simulink model "CM620A_MotAg0Meas"  (R2013b)
settings: Solver=FixedStepDiscrete  SolverMode=SingleTasking  StartTime=0.0  StopTime=1  FixedStep=0.0000625  RelTol=1e-3
undefined symbols (not defined in the file): ARCHGLBPRM_2PI_ULS_F32, COEFFTBLELMSIZE_CNT_U08, COEFFTBLSIZE_CNT_U08, CORRNTBLAGSTEPSIZE_MATRAD_F32, CORRNTBLSIDXOFFS_CNT_U16, CORRNTBLSIZE_CNT_U16, CORRNTBLSIZEMASK_CNT_U08, FLTINJ_MOTAG0MEAS_MOTCTRLMOTAG0MECL, FLTINJ_MOTAG0MEAS_TESTOK, MotAg0PrtclFlt, MOTAG0PRTCLFLTFAILSTEP_CNT_U16, MOTAG0PRTCLFLTPASSSTEP_CNT_U16, MOTAGDELTAPERCORRNPT_CNT_U16, MOTAGIDXMASK_CNT_U16, MotCtrlMotAg0ErrReg, NtcSts1, sigbuilder_block, SNSRAGMASK_CNT_U32, SNSRERRMASK_CNT_U32, SNSRERRNTCMASK_CNT_U08, SNSRVLTGFLTMASK_CNT_U32, SPIPARMASK_CNT_U32
libraries: simulink x28, FloatToFixd x1, NxtrMax x1, NxtrLim x1
(part 2 of 4)

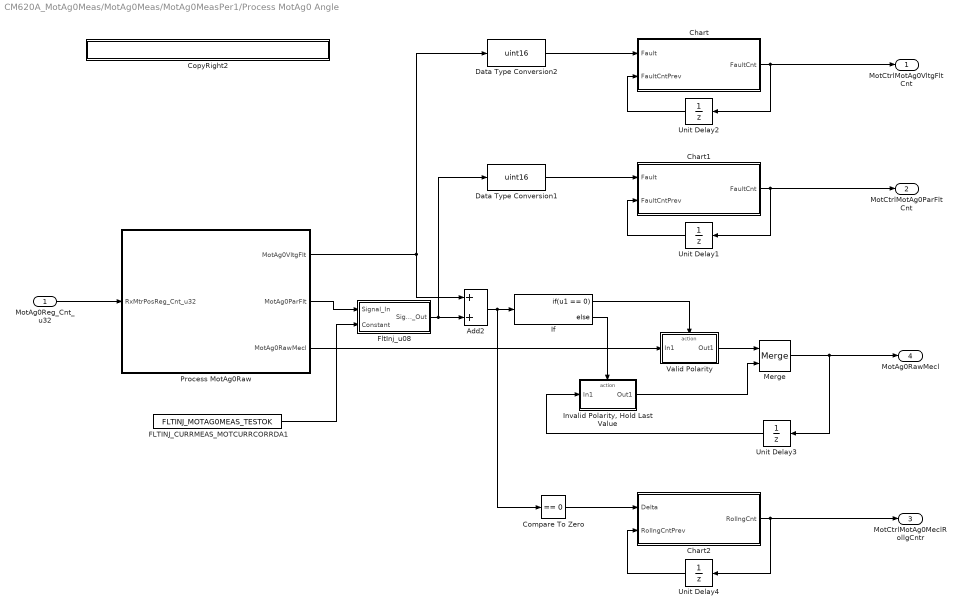
== system CM620A_MotAg0Meas/MotAg0Meas/MotAg0MeasPer1/Process MotAg0 Angle ==
  MotAg0Reg_Cnt_u32 : Inport
  Add2 : Sum  RequirementInfo={'linktype_rmi_doors' '0000c47b (/ESG Group/FDD Module Requirements/EA4 Specific/CM620A_MotAg0Meas)' '#CM620A_87' 'true' 'REQ: CM620A_87' '' } %GIDa_0b7de0f8_fdb6_403a_993a_161f92b64634
  Chart : Stateflow chart  TreatAsAtomicUnit=on
  Chart1 : Stateflow chart  TreatAsAtomicUnit=on
  Chart2 : Stateflow chart  RequirementInfo={'linktype_rmi_doors' '0000c47b (/ESG Group/FDD Module Requirements/EA4 Specific/CM620A_MotAg0Meas)' '#CM620A_107' 'true' 'REQ: CM620A_107' '' } %GIDa_4e204d7d_fe00_4721_af4a_71a94d72e207  TreatAsAtomicUnit=on
  Compare To Zero : simulink/Logic and Bit Operations/Compare To Zero  relop===  OutDataTypeStr=uint8
  CopyRight2 : Subsystem  Description=|  mask(Copyright Information){none=on}
      | Copyright info block.                                               
      |                                                                     
      | Place copyright information at the top of every subsystem in design.
      mask prompts: none "No parameters"
      mask help: Place copyright information at the top of every subsystem in design.
      mask Display:
      | NxtrConf = 'Nexteer Confidential';
      | 
      | sys = bdroot; %handle for the current model ("system")
      | first = get_param(sys,'Created');
      | first = first(end-3:end);  %year is last four digits
      | 
      | last = get_param(sys,'LastModifiedDate');
      | if isempty(last)
      |     last = datestr(now,'yyyy');
      | else
      |     last = last(end-3:end);
      | end
      | 
      | if strcmp(first,last)
      |     fprintf('%s -- Copyright %s Nexteer',NxtrConf,first)
      | else
      |     fprintf('%s -- %s%s- %s Nexteer',NxtrConf,char(169),first,last)
      | end
  Data Type Conversion1 : DataTypeConversion  OutDataTypeStr=uint16
  Data Type Conversion2 : DataTypeConversion  OutDataTypeStr=uint16
  FLTINJ_CURRMEAS_MOTCURRCORRDA1 : Constant  Value=FLTINJ_MOTAG0MEAS_TESTOK
  FltInj_u08 : Subsystem  RequirementInfo={'linktype_rmi_doors' '0000c47b (/ESG Group/FDD Module Requirements/EA4 Specific/CM620A_MotAg0Meas)' '#CM620A_111' 'true' 'REQ: CM620A_111' '' } %GIDa_ea97dbee_e66e_4906_919b_b7ed9fef212d  TreatAsAtomicUnit=on  VariantControl=FltInj_sim  mask(Fault_Injection){}
      mask help: Fault Injection is a simulation only block for EA3 programs.
  If : If  IfExpression=u1 == 0
  "Invalid Polarity, Hold Last Value" : Subsystem  TreatAsAtomicUnit=on
  Merge : Merge  RequirementInfo={'linktype_rmi_doors' '0000c47b (/ESG Group/FDD Module Requirements/EA4 Specific/CM620A_MotAg0Meas)' '#CM620A_88' 'true' 'REQ: CM620A_88' '' } %GIDa_2a6c3b81_7733_45e8_b94f_934422d25578
  Process MotAg0Raw : Subsystem  RequirementInfo={'linktype_rmi_doors' '0000c47b (/ESG Group/FDD Module Requirements/EA4 Specific/CM620A_MotAg0Meas)' '#CM620A_95' 'true' 'REQ: CM620A_95' '' ; 'linktype_rmi_doors' '0000c47b (/ESG Group/FDD Module Requirements/EA4 Specific/CM620A_MotAg0Meas)' '#CM620A_93' 'true' 'REQ: CM620A_93' '' ; 'linktype_rmi_doors' '0000c47b (/ESG Group/FDD Module Requirements/EA4 Specific/CM620A_MotAg0Meas)' '#CM620A_84' 'true' 'REQ: CM620A_84' '' ; 'linktype_rmi_doors' '0000c47b (/ESG Group/FDD Module Requirements/EA4 Specific/CM620A_MotAg0Meas)' '#CM620A_86' 'true' 'REQ: CM620A_86' '' } %GIDa_f2e2859c_06d0_4da9_b7a1_6837a8f50074
  Unit Delay1 : UnitDelay  SampleTime=-1  StateName=MotAg0ParFltCntPrev  StateMustResolveToSignalObject=on
      settings: AttributesFormatString=|
      | State Variable:
      | %<StateName>
  Unit Delay2 : UnitDelay  SampleTime=-1  StateName=MotAg0VltgFltCntPrev  StateMustResolveToSignalObject=on
      settings: AttributesFormatString=|
      | State Variable:
      | %<StateName>
  Unit Delay3 : UnitDelay  SampleTime=-1  StateName=MotAg0RawMeclPrev  StateMustResolveToSignalObject=on
      settings: AttributesFormatString=|
      | State Variable:
      | %<StateName>
  Unit Delay4 : UnitDelay  SampleTime=-1  StateName=MotAg0MeclRollgCntrPrev  StateMustResolveToSignalObject=on
      settings: AttributesFormatString=|
      | State Variable:
      | %<StateName>
  Valid Polarity : Subsystem  TreatAsAtomicUnit=on
  MotCtrlMotAg0VltgFltCnt : Outport
  MotCtrlMotAg0ParFltCnt : Outport  Port=2
  MotCtrlMotAg0MeclRollgCntr : Outport  Port=3
  MotAg0RawMecl : Outport  Port=4
  wires:
  Add2/1 -> If/1, Compare To Zero/1
  Process MotAg0Raw/1(MotAg0VltgFlt) -> Data Type Conversion2/1, Add2/1
  Unit Delay3/1 -> "Invalid Polarity, Hold Last Value"/1(In1)
  Merge/1 -> Unit Delay3/1, MotAg0RawMecl/1
  MotAg0Reg_Cnt_u32/1 -> Process MotAg0Raw/1(RxMtrPosReg_Cnt_u32)
  "Invalid Polarity, Hold Last Value"/1(Out1) -> Merge/2
  Valid Polarity/1(Out1) -> Merge/1
  If/2 -> "Invalid Polarity, Hold Last Value"/Action
  If/1 -> Valid Polarity/Action
  Process MotAg0Raw/3(MotAg0RawMecl) -> Valid Polarity/1(In1)
  Data Type Conversion2/1 -> Chart/1(Fault)
  Chart/1(FaultCnt) -> MotCtrlMotAg0VltgFltCnt/1, Unit Delay2/1
  Unit Delay2/1 -> Chart/2(FaultCntPrev)
  Data Type Conversion1/1 -> Chart1/1(Fault)
  Chart1/1(FaultCnt) -> MotCtrlMotAg0ParFltCnt/1, Unit Delay1/1
  Unit Delay1/1 -> Chart1/2(FaultCntPrev)
  Compare To Zero/1 -> Chart2/1(Delta)
  Chart2/1(RollngCnt) -> MotCtrlMotAg0MeclRollgCntr/1, Unit Delay4/1
  Unit Delay4/1 -> Chart2/2(RollngCntPrev)
  FLTINJ_CURRMEAS_MOTCURRCORRDA1/1 -> FltInj_u08/2(Constant)
  Process MotAg0Raw/2(MotAg0ParFlt) -> FltInj_u08/1(Signal_In)
  FltInj_u08/1(Signal_Out) -> Add2/2, Data Type Conversion1/1

== system CM620A_MotAg0Meas/MotAg0Meas/MotAg0MeasPer2/CopyRight2 ==

== system CM620A_MotAg0Meas/MotAg0Meas/MotAg0MeasPer2/MotAg0 Protocol Fault Operation ==
  note: Function Call Sequence Requirements
      |
      | - GetNtcQlfr shall execute after SetNtcSts
  MotAg0Err : Inport
  MotAg0ErrParFltCnt : Inport  Port=2
  MotAg0ParFltCnt : Inport  Port=3
  MotAg0VltgFltCnt : Inport  Port=4
  Atomic Subsystem : Subsystem  TreatAsAtomicUnit=on
  Constant3 : Constant  Value=MotAg0PrtclFlt
  CopyRight2 : Subsystem  Description=|  mask(Copyright Information){none=on}
      | Copyright info block.                                               
      |                                                                     
      | Place copyright information at the top of every subsystem in design.
      mask prompts: none "No parameters"
      mask help: Place copyright information at the top of every subsystem in design.
      mask Display:
      | NxtrConf = 'Nexteer Confidential';
      | 
      | sys = bdroot; %handle for the current model ("system")
      | first = get_param(sys,'Created');
      | first = first(end-3:end);  %year is last four digits
      | 
      | last = get_param(sys,'LastModifiedDate');
      | if isempty(last)
      |     last = datestr(now,'yyyy');
      | else
      |     last = last(end-3:end);
      | end
      | 
      | if strcmp(first,last)
      |     fprintf('%s -- Copyright %s Nexteer',NxtrConf,first)
      | else
      |     fprintf('%s -- %s%s- %s Nexteer',NxtrConf,char(169),first,last)
      | end
  Data store for model purposes only - don't code : DataStoreMemory  DataStoreName=NtcQlfr  ReadBeforeWriteMsg=warning  WriteAfterWriteMsg=warning  WriteAfterReadMsg=warning
  GetNtcQlfr : Subsystem  RequirementInfo={'linktype_rmi_doors' '0000c47b (/ESG Group/FDD Module Requirements/EA4 Specific/CM620A_MotAg0Meas)' '#CM620A_106' 'true' 'REQ: CM620A_106' '' } %GIDa_2788174b_a957_4dc9_a642_eff6dc86ed2e
  SetNtcSts : Subsystem
  Subsystem : Subsystem
  MotAg0Qlfr : Outport  RequirementInfo={} %GIDa_cf1cbe4f_1681_476d_80fb_f928627be900
  wires:
  MotAg0Err/1 -> Subsystem/1(MotAg0Err)
  MotAg0ErrParFltCnt/1 -> Subsystem/2(MotAg0ErrParFltCnt)
  MotAg0ParFltCnt/1 -> Subsystem/3(MotAg0ParFltCnt)
  MotAg0VltgFltCnt/1 -> Subsystem/4(MotAg0VltgFltCnt)
  Constant3/1 -> SetNtcSts/1(NtcNr), GetNtcQlfr/1(NtcNr)  "NtcNr"
  GetNtcQlfr/1(NtcQlfr) -> MotAg0Qlfr/1
  Atomic Subsystem/1(NtcSts) -> SetNtcSts/3(NtcSts)
  Atomic Subsystem/2(DebStep) -> SetNtcSts/4(DebStep)
  Subsystem/1(NtcStInfo) -> Atomic Subsystem/1(NtcStInfo), SetNtcSts/2(NtcStInfo)  "ParamByte"

== system CM620A_MotAg0Meas/MotAg0Meas/MotAg0MeasPer2/Process ErrorReg and DieRevCtr ==
  MotAg0ErrReg : Inport  OutDataTypeStr=uint32
  CopyRight2 : Subsystem  Description=|  mask(Copyright Information){none=on}
      | Copyright info block.                                               
      |                                                                     
      | Place copyright information at the top of every subsystem in design.
      mask prompts: none "No parameters"
      mask help: Place copyright information at the top of every subsystem in design.
      mask Display:
      | NxtrConf = 'Nexteer Confidential';
      | 
      | sys = bdroot; %handle for the current model ("system")
      | first = get_param(sys,'Created');
      | first = first(end-3:end);  %year is last four digits
      | 
      | last = get_param(sys,'LastModifiedDate');
      | if isempty(last)
      |     last = datestr(now,'yyyy');
      | else
      |     last = last(end-3:end);
      | end
      | 
      | if strcmp(first,last)
      |     fprintf('%s -- Copyright %s Nexteer',NxtrConf,first)
      | else
      |     fprintf('%s -- %s%s- %s Nexteer',NxtrConf,char(169),first,last)
      | end
  Process MotAg0RawErr : Subsystem  RequirementInfo={'linktype_rmi_doors' '0000c47b (/ESG Group/FDD Module Requirements/EA4 Specific/CM620A_MotAg0Meas)' '#CM620A_93' 'true' 'REQ: CM620A_93' '' } %GIDa_05fef35d_e67f_443b_a4d0_6048385f8050
  MotAg0Err : Outport  OutDataTypeStr=uint8
  MotAg0ErrParFltCnt : Outport  Port=2
  wires:
  MotAg0ErrReg/1 -> Process MotAg0RawErr/1(MotAg0ErrReg)
  Process MotAg0RawErr/1(MotAg0ErrParFltCnt) -> MotAg0ErrParFltCnt/1
  Process MotAg0RawErr/2(MotAg0Err) -> MotAg0Err/1

== system CM620A_MotAg0Meas/MotAg0Meas/MotAg0MeasInit1/Compute Correction Table/CopyRight2 ==

== system CM620A_MotAg0Meas/MotAg0Meas/MotAg0MeasInit1/Compute Correction Table/MotAg0CoeffTbl_GetErrorStatus ==
  note: 0 simulated for modeling purposes,
      | actual value returned by NVM.  Non-zero return indicates
      | failure in storage/retrievial of NVM.
  Constant : Constant  Value=0
  CopyRight2 : Subsystem  Description=|  mask(Copyright Information){none=on}
      | Copyright info block.                                               
      |                                                                     
      | Place copyright information at the top of every subsystem in design.
      mask prompts: none "No parameters"
      mask help: Place copyright information at the top of every subsystem in design.
      mask Display:
      | NxtrConf = 'Nexteer Confidential';
      | 
      | sys = bdroot; %handle for the current model ("system")
      | first = get_param(sys,'Created');
      | first = first(end-3:end);  %year is last four digits
      | 
      | last = get_param(sys,'LastModifiedDate');
      | if isempty(last)
      |     last = datestr(now,'yyyy');
      | else
      |     last = last(end-3:end);
      | end
      | 
      | if strcmp(first,last)
      |     fprintf('%s -- Copyright %s Nexteer',NxtrConf,first)
      | else
      |     fprintf('%s -- %s%s- %s Nexteer',NxtrConf,char(169),first,last)
      | end
  RequestResultPtr : Outport
  wires:
  Constant/1 -> RequestResultPtr/1

== system CM620A_MotAg0Meas/MotAg0Meas/MotAg0MeasInit1/Compute Correction Table/NVM NOK ==
  note: In the event of a NVM failure
      | set the correction table to 0
  Action Port : ActionPort  ActionType=else
  Constant1 : Constant  Value=CORRNTBLSIZE_CNT_U16
  CopyRight2 : Subsystem  Description=|  mask(Copyright Information){none=on}
      | Copyright info block.                                               
      |                                                                     
      | Place copyright information at the top of every subsystem in design.
      mask prompts: none "No parameters"
      mask help: Place copyright information at the top of every subsystem in design.
      mask Display:
      | NxtrConf = 'Nexteer Confidential';
      | 
      | sys = bdroot; %handle for the current model ("system")
      | first = get_param(sys,'Created');
      | first = first(end-3:end);  %year is last four digits
      | 
      | last = get_param(sys,'LastModifiedDate');
      | if isempty(last)
      |     last = datestr(now,'yyyy');
      | else
      |     last = last(end-3:end);
      | end
      | 
      | if strcmp(first,last)
      |     fprintf('%s -- Copyright %s Nexteer',NxtrConf,first)
      | else
      |     fprintf('%s -- %s%s- %s Nexteer',NxtrConf,char(169),first,last)
      | end
  Zero out correction table : Subsystem  TreatAsAtomicUnit=on
  wires:
  Constant1/1 -> Zero out correction table/1(N)

== system CM620A_MotAg0Meas/MotAg0Meas/MotAg0MeasInit1/Compute Correction Table/NVM Ok ==
  Action Port : ActionPort  ActionType=then
  Calculate Correction Table : Subsystem  Priority=100  TreatAsAtomicUnit=on
      settings: AttributesFormatString=|
      | Priority:
      | %<Priority>
  Configure Coefficients : Subsystem  Priority=10  TreatAsAtomicUnit=on
      settings: AttributesFormatString=|
      | Priority:
      | %<Priority>
  CopyRight2 : Subsystem  Description=|  mask(Copyright Information){none=on}
      | Copyright info block.                                               
      |                                                                     
      | Place copyright information at the top of every subsystem in design.
      mask prompts: none "No parameters"
      mask help: Place copyright information at the top of every subsystem in design.
      mask Display:
      | NxtrConf = 'Nexteer Confidential';
      | 
      | sys = bdroot; %handle for the current model ("system")
      | first = get_param(sys,'Created');
      | first = first(end-3:end);  %year is last four digits
      | 
      | last = get_param(sys,'LastModifiedDate');
      | if isempty(last)
      |     last = datestr(now,'yyyy');
      | else
      |     last = last(end-3:end);
      | end
      | 
      | if strcmp(first,last)
      |     fprintf('%s -- Copyright %s Nexteer',NxtrConf,first)
      | else
      |     fprintf('%s -- %s%s- %s Nexteer',NxtrConf,char(169),first,last)
      | end

== system CM620A_MotAg0Meas/MotAg0Meas/MotAg0MeasInit1/Initialize CSIH Registers/CopyRight2 ==

== system CM620A_MotAg0Meas/MotAg0Meas/MotAg0MeasPer1/Compensate MechMtrPos1/CopyRight2 ==

== system CM620A_MotAg0Meas/MotAg0Meas/MotAg0MeasPer1/FltInj_u0p16/Copyright1 ==

== system CM620A_MotAg0Meas/MotAg0Meas/MotAg0MeasPer1/GetRefTmr1MicroSec32bit/CopyRight2 ==

== system CM620A_MotAg0Meas/MotAg0Meas/MotAg0MeasPer1/Process MotAg0 Angle/CopyRight2 ==

== system CM620A_MotAg0Meas/MotAg0Meas/MotAg0MeasPer1/Process MotAg0 Angle/FltInj_u08 ==
  note: This block requires no modification by FDD author.
      |
      | This block does not actually simulate any fault injection.  It is simply a pass-thru.
      |
      | The Constant port (#2) simply terminates its signal, but we are trying to force the FDD author
      | to properly use the FltInjectionLocType enumeration in FDD model.
  note: EA4.x Fault Injection
  Signal_In : Inport
  Constant : Inport  Port=2
  CopyRight2 : Subsystem  Description=|  mask(Copyright Information){none=on}
      | Copyright info block.                                               
      |                                                                     
      | Place copyright information at the top of every subsystem in design.
      mask prompts: none "No parameters"
      mask help: Place copyright information at the top of every subsystem in design.
      mask Display:
      | NxtrConf = 'Nexteer Confidential';
      | 
      | sys = bdroot; %handle for the current model ("system")
      | first = get_param(sys,'Created');
      | first = first(end-3:end);  %year is last four digits
      | 
      | last = get_param(sys,'LastModifiedDate');
      | if isempty(last)
      |     last = datestr(now,'yyyy');
      | else
      |     last = last(end-3:end);
      | end
      | 
      | if strcmp(first,last)
      |     fprintf('%s -- Copyright %s Nexteer',NxtrConf,first)
      | else
      |     fprintf('%s -- %s%s- %s Nexteer',NxtrConf,char(169),first,last)
      | end
  Terminator : Terminator
  Signal_Out : Outport
  wires:
  Signal_In/1 -> Signal_Out/1
  Constant/1 -> Terminator/1

== system CM620A_MotAg0Meas/MotAg0Meas/MotAg0MeasPer1/Process MotAg0 Angle/Invalid Polarity, Hold Last Value ==
  In1 : Inport
  Action Port : ActionPort  ActionType=else
  Out1 : Outport
  wires:
  In1/1 -> Out1/1

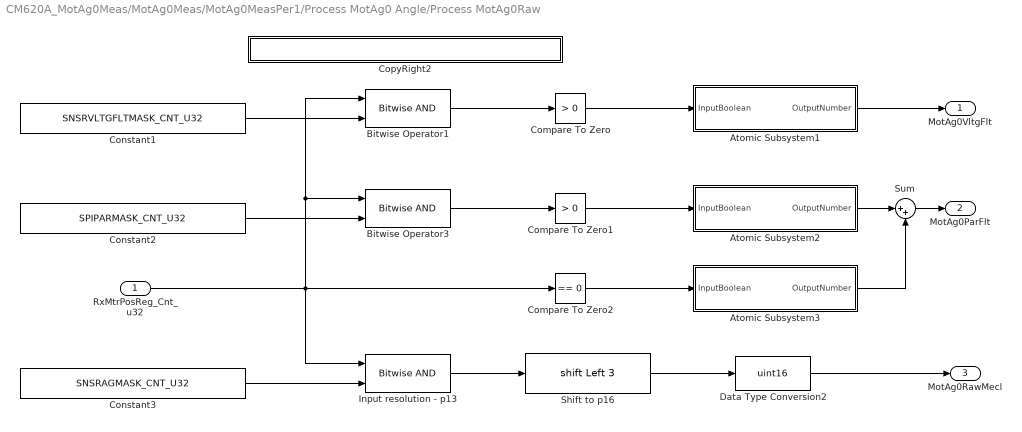
== system CM620A_MotAg0Meas/MotAg0Meas/MotAg0MeasPer1/Process MotAg0 Angle/Process MotAg0Raw ==
  RxMtrPosReg_Cnt_u32 : Inport  OutDataTypeStr=uint32
  Atomic Subsystem1 : Subsystem  TreatAsAtomicUnit=on
  Atomic Subsystem2 : Subsystem  TreatAsAtomicUnit=on
  Atomic Subsystem3 : Subsystem  TreatAsAtomicUnit=on
  Bitwise Operator1 : simulink/Logic and Bit Operations/Bitwise Operator  logicop=AND  UseBitMask=off  NumInputPorts=2  BitMask=SNSRVLTGFLTMASK_CNT_U32  BitMaskRealWorld=Stored Integer
  Bitwise Operator3 : simulink/Logic and Bit Operations/Bitwise Operator  logicop=AND  UseBitMask=off  NumInputPorts=2  BitMask=SPIPARMASK_CNT_U32  BitMaskRealWorld=Stored Integer
  Compare To Zero : simulink/Logic and Bit Operations/Compare To Zero  relop=>  OutDataTypeStr=boolean
  Compare To Zero1 : simulink/Logic and Bit Operations/Compare To Zero  relop=>  OutDataTypeStr=boolean
  Compare To Zero2 : simulink/Logic and Bit Operations/Compare To Zero  relop===  OutDataTypeStr=boolean
  Constant1 : Constant  Value=SNSRVLTGFLTMASK_CNT_U32
  Constant2 : Constant  Value=SPIPARMASK_CNT_U32
  Constant3 : Constant  Value=SNSRAGMASK_CNT_U32
  CopyRight2 : Subsystem  Description=|  mask(Copyright Information){none=on}
      | Copyright info block.                                               
      |                                                                     
      | Place copyright information at the top of every subsystem in design.
      mask prompts: none "No parameters"
      mask help: Place copyright information at the top of every subsystem in design.
      mask Display:
      | NxtrConf = 'Nexteer Confidential';
      | 
      | sys = bdroot; %handle for the current model ("system")
      | first = get_param(sys,'Created');
      | first = first(end-3:end);  %year is last four digits
      | 
      | last = get_param(sys,'LastModifiedDate');
      | if isempty(last)
      |     last = datestr(now,'yyyy');
      | else
      |     last = last(end-3:end);
      | end
      | 
      | if strcmp(first,last)
      |     fprintf('%s -- Copyright %s Nexteer',NxtrConf,first)
      | else
      |     fprintf('%s -- %s%s- %s Nexteer',NxtrConf,char(169),first,last)
      | end
  Data Type Conversion2 : DataTypeConversion  OutDataTypeStr=uint16
  Input resolution - p13 : simulink/Logic and Bit Operations/Bitwise Operator  logicop=AND  UseBitMask=off  NumInputPorts=2  BitMask=SNSRAGMASK_CNT_U32  BitMaskRealWorld=Stored Integer
  Shift to p16 : ArithShift  BitShiftNumber=3  BitShiftDirection=Left
  Sum : Sum  Inputs=|++
  MotAg0VltgFlt : Outport
  MotAg0ParFlt : Outport  Port=2
  MotAg0RawMecl : Outport  Port=3
  wires:
  Compare To Zero/1 -> Atomic Subsystem1/1(InputBoolean)
  Bitwise Operator1/1 -> Compare To Zero/1
  Bitwise Operator3/1 -> Compare To Zero1/1
  RxMtrPosReg_Cnt_u32/1 -> Input resolution - p13/1, Compare To Zero2/1, Bitwise Operator1/1, Bitwise Operator3/1
  Compare To Zero1/1 -> Atomic Subsystem2/1(InputBoolean)
  Input resolution - p13/1 -> Shift to p16/1
  Data Type Conversion2/1 -> MotAg0RawMecl/1
  Atomic Subsystem2/1(OutputNumber) -> Sum/1
  Atomic Subsystem1/1(OutputNumber) -> MotAg0VltgFlt/1
  Shift to p16/1 -> Data Type Conversion2/1
  Compare To Zero2/1 -> Atomic Subsystem3/1(InputBoolean)
  Atomic Subsystem3/1(OutputNumber) -> Sum/2
  Sum/1 -> MotAg0ParFlt/1
  Constant3/1 -> Input resolution - p13/2
  Constant2/1 -> Bitwise Operator3/2
  Constant1/1 -> Bitwise Operator1/2

== system CM620A_MotAg0Meas/MotAg0Meas/MotAg0MeasPer1/Process MotAg0 Angle/Valid Polarity ==
  In1 : Inport
  Action Port : ActionPort  ActionType=then
  Out1 : Outport
  wires:
  In1/1 -> Out1/1

== system CM620A_MotAg0Meas/MotAg0Meas/MotAg0MeasPer2/MotAg0 Protocol Fault Operation/Atomic Subsystem ==
  NtcStInfo : Inport  OutDataTypeStr=uint8
  CopyRight2 : Subsystem  Description=|  mask(Copyright Information){none=on}
      | Copyright info block.                                               
      |                                                                     
      | Place copyright information at the top of every subsystem in design.
      mask prompts: none "No parameters"
      mask help: Place copyright information at the top of every subsystem in design.
      mask Display:
      | NxtrConf = 'Nexteer Confidential';
      | 
      | sys = bdroot; %handle for the current model ("system")
      | first = get_param(sys,'Created');
      | first = first(end-3:end);  %year is last four digits
      | 
      | last = get_param(sys,'LastModifiedDate');
      | if isempty(last)
      |     last = datestr(now,'yyyy');
      | else
      |     last = last(end-3:end);
      | end
      | 
      | if strcmp(first,last)
      |     fprintf('%s -- Copyright %s Nexteer',NxtrConf,first)
      | else
      |     fprintf('%s -- %s%s- %s Nexteer',NxtrConf,char(169),first,last)
      | end
  If : If
  Merge : Merge
  Merge1 : Merge
  N Step : Subsystem  RequirementInfo={'linktype_rmi_doors' '0000c47b (/ESG Group/FDD Module Requirements/EA4 Specific/CM620A_MotAg0Meas)' '#CM620A_31' 'true' 'REQ: CM620A_31' '' } %GIDa_a1ed8da0_4c35_4cb0_a2c6_08587c652881  TreatAsAtomicUnit=on
  P Step : Subsystem  TreatAsAtomicUnit=on
  NtcSts : Outport
  DebStep : Outport  Port=2  OutDataTypeStr=uint16
  wires:
  NtcStInfo/1 -> If/1
  If/1 -> P Step/Action
  If/2 -> N Step/Action
  Merge/1 -> DebStep/1
  P Step/1(NtcSts) -> Merge1/1
  N Step/1(NtcSts) -> Merge1/2
  Merge1/1 -> NtcSts/1
  P Step/2(DebStep) -> Merge/1
  N Step/2(DebStep) -> Merge/2

== system CM620A_MotAg0Meas/MotAg0Meas/MotAg0MeasPer2/MotAg0 Protocol Fault Operation/CopyRight2 ==

== system CM620A_MotAg0Meas/MotAg0Meas/MotAg0MeasPer2/MotAg0 Protocol Fault Operation/GetNtcQlfr ==
  NtcNr : Inport
  CopyRight2 : Subsystem  Description=|  mask(Copyright Information){none=on}
      | Copyright info block.                                               
      |                                                                     
      | Place copyright information at the top of every subsystem in design.
      mask prompts: none "No parameters"
      mask help: Place copyright information at the top of every subsystem in design.
      mask Display:
      | NxtrConf = 'Nexteer Confidential';
      | 
      | sys = bdroot; %handle for the current model ("system")
      | first = get_param(sys,'Created');
      | first = first(end-3:end);  %year is last four digits
      | 
      | last = get_param(sys,'LastModifiedDate');
      | if isempty(last)
      |     last = datestr(now,'yyyy');
      | else
      |     last = last(end-3:end);
      | end
      | 
      | if strcmp(first,last)
      |     fprintf('%s -- Copyright %s Nexteer',NxtrConf,first)
      | else
      |     fprintf('%s -- %s%s- %s Nexteer',NxtrConf,char(169),first,last)
      | end
  Data Store Read : DataStoreRead  DataStoreName=NtcQlfr
  Terminator : Terminator
  NtcQlfr : Outport
  wires:
  NtcNr/1 -> Terminator/1
  Data Store Read/1 -> NtcQlfr/1

== system CM620A_MotAg0Meas/MotAg0Meas/MotAg0MeasPer2/MotAg0 Protocol Fault Operation/SetNtcSts ==
  note: Note:
      |
      | - "ISO Fault Debounce Design" Simulink block intent to use here for Simulation purpose only. Do not Code this block
  NtcNr : Inport
  NtcStInfo : Inport  Port=2
  NtcSts : Inport  Port=3  OutDataTypeStr=Enum: NtcSts1
  DebStep : Inport  Port=4
  CopyRight2 : Subsystem  Description=|  mask(Copyright Information){none=on}
      | Copyright info block.                                               
      |                                                                     
      | Place copyright information at the top of every subsystem in design.
      mask prompts: none "No parameters"
      mask help: Place copyright information at the top of every subsystem in design.
      mask Display:
      | NxtrConf = 'Nexteer Confidential';
      | 
      | sys = bdroot; %handle for the current model ("system")
      | first = get_param(sys,'Created');
      | first = first(end-3:end);  %year is last four digits
      | 
      | last = get_param(sys,'LastModifiedDate');
      | if isempty(last)
      |     last = datestr(now,'yyyy');
      | else
      |     last = last(end-3:end);
      | end
      | 
      | if strcmp(first,last)
      |     fprintf('%s -- Copyright %s Nexteer',NxtrConf,first)
      | else
      |     fprintf('%s -- %s%s- %s Nexteer',NxtrConf,char(169),first,last)
      | end
  Data Store Write : DataStoreWrite  DataStoreName=NtcQlfr
  Data Type Conversion1 : DataTypeConversion  OutDataTypeStr=uint8
  Ground : Ground
  ISO Fault Debounce Design : Stateflow chart  TreatAsAtomicUnit=on
      settings: AttributesFormatString=|
      | Simulation Purpose Only.
      | Do Not Code this block
      | Diagnostic Manager Owns this requirement
  Scope1 : Scope  NumInputPorts=4
      settings: YMin=-5~-5~-5~-5  YMax=5~5~5~5  SaveName=ScopeData5
  Terminator : Terminator
  Terminator1 : Terminator
  wires:
  NtcStInfo/1 -> Scope1/4, Terminator1/1
  NtcNr/1 -> Terminator/1
  NtcSts/1 -> Data Type Conversion1/1
  DebStep/1 -> ISO Fault Debounce Design/2(DebStep), Scope1/2
  ISO Fault Debounce Design/1(Qualifier) -> Scope1/3, Data Store Write/1
  Ground/1 -> ISO Fault Debounce Design/3(SvcClr)
  Data Type Conversion1/1 -> ISO Fault Debounce Design/1(NtcSts), Scope1/1

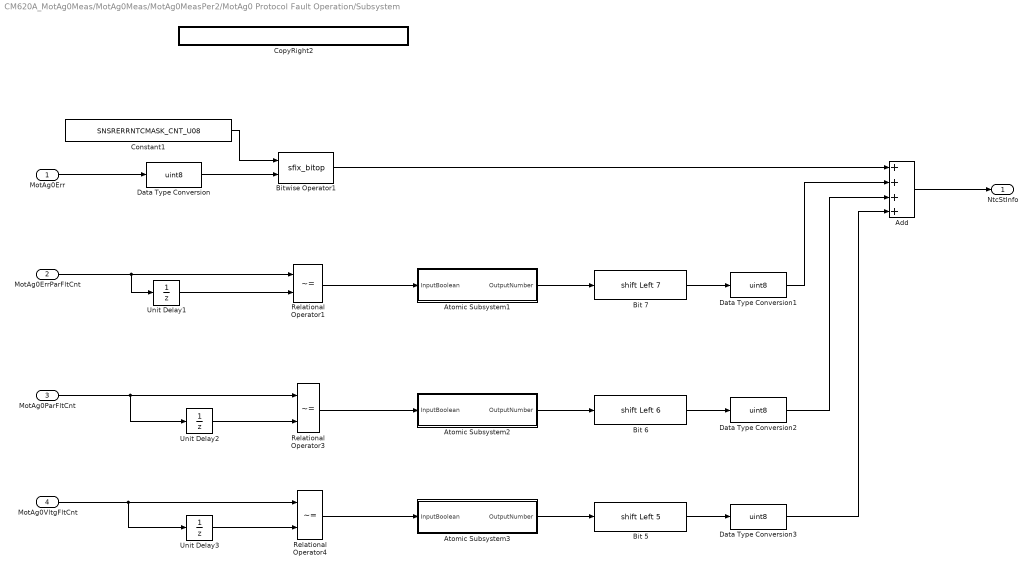
== system CM620A_MotAg0Meas/MotAg0Meas/MotAg0MeasPer2/MotAg0 Protocol Fault Operation/Subsystem ==
  MotAg0Err : Inport  RequirementInfo={'linktype_rmi_doors' '0000c47b (/ESG Group/FDD Module Requirements/EA4 Specific/CM620A_MotAg0Meas)' '#CM620A_98' 'true' 'REQ: CM620A_98' '' ; 'linktype_rmi_doors' '0000c47b (/ESG Group/FDD Module Requirements/EA4 Specific/CM620A_MotAg0Meas)' '#CM620A_99' 'true' 'REQ: CM620A_99' '' ; 'linktype_rmi_doors' '0000c47b (/ESG Group/FDD Module Requirements/EA4 Specific/CM620A_MotAg0Meas)' '#CM620A_100' 'true' 'REQ: CM620A_100' '' } %GIDa_6edd1ae9_9c74_4544_bf40_7d9417b836a7
  MotAg0ErrParFltCnt : Inport  Port=2
  MotAg0ParFltCnt : Inport  Port=3
  MotAg0VltgFltCnt : Inport  Port=4
  Add : Sum  Inputs=++++
  Atomic Subsystem1 : Subsystem  TreatAsAtomicUnit=on
  Atomic Subsystem2 : Subsystem  TreatAsAtomicUnit=on
  Atomic Subsystem3 : Subsystem  TreatAsAtomicUnit=on
  Bit 5 : ArithShift  BitShiftNumber=5  BitShiftDirection=Left
  Bit 6 : ArithShift  BitShiftNumber=6  BitShiftDirection=Left
  Bit 7 : ArithShift  BitShiftNumber=7  BitShiftDirection=Left
  Bitwise Operator1 : S-Function  RequirementInfo={'linktype_rmi_doors' '0000c47b (/ESG Group/FDD Module Requirements/EA4 Specific/CM620A_MotAg0Meas)' '#CM620A_91' 'true' 'REQ: CM620A_91' '' ; 'linktype_rmi_doors' '0000c47b (/ESG Group/FDD Module Requirements/EA4 Specific/CM620A_MotAg0Meas)' '#CM620A_98' 'true' 'REQ: CM620A_98' '' ; 'linktype_rmi_doors' '0000c47b (/ESG Group/FDD Module Requirements/EA4 Specific/CM620A_MotAg0Meas)' '#CM620A_99' 'true' 'REQ: CM620A_99' '' ; 'linktype_rmi_doors' '0000c47b (/ESG Group/FDD Module Requirements/EA4 Specific/CM620A_MotAg0Meas)' '#CM620A_100' 'true' 'REQ: CM620A_100' '' } %GIDa_5c9d0cb2_6ffb_4aa7_875c_2abe2058166d  FunctionName=sfix_bitop  Parameters=UseBitMask,NumInputPorts,BitMask,BitMaskRealWorld,logicop  EnableBusSupport=off  mask(Bitwise Operator){logicop=AND, UseBitMask=off, NumInputPorts=2, BitMask=SNSRERRNTCMASK_CNT_U08, BitMaskRealWorld=Stored Integer}
      mask prompts: logicop "Operator:"; UseBitMask "Use bit mask ..."; NumInputPorts "Number of input ports:"; BitMask "Bit Mask"; BitMaskRealWorld "Treat mask as:"
      mask help: Perform the specified bitwise operation on the inputs. The output data type should represent zero exactly.
      mask init:
      | str = '';
      | if UseBitMask
      |   [m,n] = size(BitMask);
      |   if ischar(BitMask)
      |     len = m;
      |     n = 1;
      |   else
      |     len = m * n;
      |   end
      |   internalBitMask = zeros(m,n);
      |   if isnumeric(BitMask)
      |     for i=1:len,
      |       internalBitMask(i) = BitMask(i);
      |     end
      |   elseif ischar(BitMask)
      |     for i=1:m,
      |       internalBitMask(i) = hex2dec(BitMask(i,:));
      |     end
      |   elseif iscell(BitMask)
      |     for i=1:len,
      |       if isnumeric( BitMask{i} )
      |         internalBitMask(i) = BitMask{i};
      |       elseif ischar( BitMask{i} )
      |         internalBitMask(i) = hex2dec(BitMask{i});
      |       else
      |         errordlg(['Data type is not supported at cell item ', num2str(i) ]);
      |       end
      |     end
      |   end
      |   BitMask = internalBitMask;
      |   for i=1:len
      |     if BitMask(i) > (2^52)-1
      |       error(DAStudio.message('Simulink:blocks:BitMaskWordLengthTooLarge')); 
      |     end
      |   end 
      |   if len == 1
      |      if BitMaskRealWorld == 1 || BitMask(1) < 0
      |        str=num2str(BitMask(1));
      |      else
      |        str=['0x',dec2hex(floor(BitMask(1)))];
      |      end
      |   else
      |      str='Masks';
      |   end
      | else
      |   BitMask = 0;
      |   str='';
      | end
      mask TypeOptions logicop: AND | OR | NAND | NOR | XOR | NOT
      mask Callback logicop: fixptdialog(gcbh)
      mask Callback UseBitMask: fixptdialog(gcbh)
      mask TypeOptions BitMaskRealWorld: Real World Value | Stored Integer
      mask Display: fprintf(['Bitwise\n',logicop,'\n',str])
  Constant1 : Constant  Value=SNSRERRNTCMASK_CNT_U08
  CopyRight2 : Subsystem  Description=|  mask(Copyright Information){none=on}
      | Copyright info block.                                               
      |                                                                     
      | Place copyright information at the top of every subsystem in design.
      mask prompts: none "No parameters"
      mask help: Place copyright information at the top of every subsystem in design.
      mask Display:
      | NxtrConf = 'Nexteer Confidential';
      | 
      | sys = bdroot; %handle for the current model ("system")
      | first = get_param(sys,'Created');
      | first = first(end-3:end);  %year is last four digits
      | 
      | last = get_param(sys,'LastModifiedDate');
      | if isempty(last)
      |     last = datestr(now,'yyyy');
      | else
      |     last = last(end-3:end);
      | end
      | 
      | if strcmp(first,last)
      |     fprintf('%s -- Copyright %s Nexteer',NxtrConf,first)
      | else
      |     fprintf('%s -- %s%s- %s Nexteer',NxtrConf,char(169),first,last)
      | end
  Data Type Conversion{,1..3} (4 alike) : DataTypeConversion  OutDataTypeStr=uint8
  Relational Operator1 : RelationalOperator  Operator=~=  OutDataTypeStr=boolean
  Relational Operator3 : RelationalOperator  Operator=~=  OutDataTypeStr=boolean
  Relational Operator4 : RelationalOperator  Operator=~=  OutDataTypeStr=boolean
  Unit Delay1 : UnitDelay  SampleTime=-1  StateName=MotAg0ErrParFltNtcStInfoCntPrev  StateMustResolveToSignalObject=on
      settings: AttributesFormatString=|
      | State Variable:
      | %<StateName>
  Unit Delay2 : UnitDelay  SampleTime=-1  StateName=MotAg0ParFltNtcStInfoCntPrev  StateMustResolveToSignalObject=on
      settings: AttributesFormatString=|
      | State Variable:
      | %<StateName>
  Unit Delay3 : UnitDelay  SampleTime=-1  StateName=MotAg0VltgFltNtcStInfoCntPrev  StateMustResolveToSignalObject=on
      settings: AttributesFormatString=|
      | State Variable:
      | %<StateName>
  NtcStInfo : Outport
  wires:
  Add/1 -> NtcStInfo/1
  Relational Operator3/1 -> Atomic Subsystem2/1(InputBoolean)
  MotAg0ParFltCnt/1 -> Unit Delay2/1, Relational Operator3/1
  Unit Delay1/1 -> Relational Operator1/2
  MotAg0ErrParFltCnt/1 -> Unit Delay1/1, Relational Operator1/1
  MotAg0Err/1 -> Data Type Conversion/1
  Relational Operator4/1 -> Atomic Subsystem3/1(InputBoolean)
  Unit Delay3/1 -> Relational Operator4/2
  MotAg0VltgFltCnt/1 -> Unit Delay3/1, Relational Operator4/1
  Bitwise Operator1/1 -> Add/1
  Unit Delay2/1 -> Relational Operator3/2
  Relational Operator1/1 -> Atomic Subsystem1/1(InputBoolean)
  Atomic Subsystem1/1(OutputNumber) -> Bit 7/1
  Atomic Subsystem2/1(OutputNumber) -> Bit 6/1
  Atomic Subsystem3/1(OutputNumber) -> Bit 5/1
  Data Type Conversion3/1 -> Add/4
  Data Type Conversion2/1 -> Add/3
  Data Type Conversion1/1 -> Add/2
  Bit 5/1 -> Data Type Conversion3/1
  Bit 6/1 -> Data Type Conversion2/1
  Bit 7/1 -> Data Type Conversion1/1
  Constant1/1 -> Bitwise Operator1/1
  Data Type Conversion/1 -> Bitwise Operator1/2

== system CM620A_MotAg0Meas/MotAg0Meas/MotAg0MeasPer2/Process ErrorReg and DieRevCtr/CopyRight2 ==

== system CM620A_MotAg0Meas/MotAg0Meas/MotAg0MeasPer2/Process ErrorReg and DieRevCtr/Process MotAg0RawErr ==
  MotAg0ErrReg : Inport
  Chart1 : Stateflow chart  TreatAsAtomicUnit=on
  CopyRight2 : Subsystem  Description=|  mask(Copyright Information){none=on}
      | Copyright info block.                                               
      |                                                                     
      | Place copyright information at the top of every subsystem in design.
      mask prompts: none "No parameters"
      mask help: Place copyright information at the top of every subsystem in design.
      mask Display:
      | NxtrConf = 'Nexteer Confidential';
      | 
      | sys = bdroot; %handle for the current model ("system")
      | first = get_param(sys,'Created');
      | first = first(end-3:end);  %year is last four digits
      | 
      | last = get_param(sys,'LastModifiedDate');
      | if isempty(last)
      |     last = datestr(now,'yyyy');
      | else
      |     last = last(end-3:end);
      | end
      | 
      | if strcmp(first,last)
      |     fprintf('%s -- Copyright %s Nexteer',NxtrConf,first)
      | else
      |     fprintf('%s -- %s%s- %s Nexteer',NxtrConf,char(169),first,last)
      | end
  Data Type Conversion1 : DataTypeConversion  OutDataTypeStr=uint16
  If : If  IfExpression=u1 == 0
  "Invalid Polarity, Hold Last Value" : Subsystem  TreatAsAtomicUnit=on
  Merge : Merge
  Process MotAg0RawErr : Subsystem
  Unit Delay1 : UnitDelay  SampleTime=-1  StateName=MotAg0ErrParFltCntPrev  StateMustResolveToSignalObject=on
      settings: AttributesFormatString=|
      | State Variable:
      | %<StateName>
  Unit Delay3 : UnitDelay  SampleTime=-1  StateName=MotAg0ErrPrev  StateMustResolveToSignalObject=on
      settings: AttributesFormatString=|
      | State Variable:
      | %<StateName>
  Valid Polarity : Subsystem  TreatAsAtomicUnit=on
  MotAg0ErrParFltCnt : Outport
  MotAg0Err : Outport  Port=2  OutDataTypeStr=uint8
  wires:
  Process MotAg0RawErr/1(MotAg0ErrParFlt) -> If/1, Data Type Conversion1/1
  Unit Delay3/1 -> "Invalid Polarity, Hold Last Value"/1(In1)
  Merge/1 -> Unit Delay3/1, MotAg0Err/1
  MotAg0ErrReg/1 -> Process MotAg0RawErr/1(MotAg0ErrReg)
  "Invalid Polarity, Hold Last Value"/1(Out1) -> Merge/2
  Valid Polarity/1(Out1) -> Merge/1
  If/2 -> "Invalid Polarity, Hold Last Value"/Action
  If/1 -> Valid Polarity/Action
  Process MotAg0RawErr/2(MotAg0Err) -> Valid Polarity/1(In1)
  Data Type Conversion1/1 -> Chart1/1(Fault)
  Chart1/1(FaultCnt) -> MotAg0ErrParFltCnt/1, Unit Delay1/1
  Unit Delay1/1 -> Chart1/2(FaultCntPrev)

== system CM620A_MotAg0Meas/MotAg0Meas/MotAg0MeasInit1/Compute Correction Table/MotAg0CoeffTbl_GetErrorStatus/CopyRight2 ==

== system CM620A_MotAg0Meas/MotAg0Meas/MotAg0MeasInit1/Compute Correction Table/NVM NOK/CopyRight2 ==

== system CM620A_MotAg0Meas/MotAg0Meas/MotAg0MeasInit1/Compute Correction Table/NVM NOK/Zero out correction table ==
  N : Inport
  Assignment : Assignment  IndexMode=Zero-based  IndexOptions=Index vector (port)  Indices=1  OutputSizes=1
  CopyRight2 : Subsystem  Description=|  mask(Copyright Information){none=on}
      | Copyright info block.                                               
      |                                                                     
      | Place copyright information at the top of every subsystem in design.
      mask prompts: none "No parameters"
      mask help: Place copyright information at the top of every subsystem in design.
      mask Display:
      | NxtrConf = 'Nexteer Confidential';
      | 
      | sys = bdroot; %handle for the current model ("system")
      | first = get_param(sys,'Created');
      | first = first(end-3:end);  %year is last four digits
      | 
      | last = get_param(sys,'LastModifiedDate');
      | if isempty(last)
      |     last = datestr(now,'yyyy');
      | else
      |     last = last(end-3:end);
      | end
      | 
      | if strcmp(first,last)
      |     fprintf('%s -- Copyright %s Nexteer',NxtrConf,first)
      | else
      |     fprintf('%s -- %s%s- %s Nexteer',NxtrConf,char(169),first,last)
      | end
  Data Store Read : DataStoreRead  DataStoreName=MotAg0CorrnTbl
  Data Store Write : DataStoreWrite  DataStoreName=MotAg0CorrnTbl
  For Iterator : ForIterator  ResetStates=reset  IterationSource=external  IndexMode=Zero-based  IterationVariableDataType=int16
  Zero : Constant  Value=0  OutDataTypeStr=int8
  wires:
  For Iterator/1 -> Assignment/3
  N/1 -> For Iterator/1
  Data Store Read/1 -> Assignment/1
  Assignment/1 -> Data Store Write/1
  Zero/1 -> Assignment/2

== system CM620A_MotAg0Meas/MotAg0Meas/MotAg0MeasInit1/Compute Correction Table/NVM Ok/Calculate Correction Table ==
  Build Wave : Subsystem  RequirementInfo="{'linktype_rmi_doors' '0000c47b (/ESG Group/FDD Module Requirements/EA4 Specific/CM620A_MotAg0Meas)' '#CM620A_117' 'true' 'REQ:  CM620A_117' '' } %GIDa_19855d62_ec05_463e_a9a2_14f8ab2007cc"  TreatAsAtomicUnit=on
  Change Correction Coordinate : Subsystem  RequirementInfo="{'linktype_rmi_doors' '0000c47b (/ESG Group/FDD Module Requirements/EA4 Specific/CM620A_MotAg0Meas)' '#CM620A_119' 'true' 'REQ:  CM620A_119' '' } %GIDa_1396db65_605a_4217_b88a_fb06c15f8b0f"  TreatAsAtomicUnit=on
  CopyRight2 : Subsystem  Description=|  mask(Copyright Information){none=on}
      | Copyright info block.                                               
      |                                                                     
      | Place copyright information at the top of every subsystem in design.
      mask prompts: none "No parameters"
      mask help: Place copyright information at the top of every subsystem in design.
      mask Display:
      | NxtrConf = 'Nexteer Confidential';
      | 
      | sys = bdroot; %handle for the current model ("system")
      | first = get_param(sys,'Created');
      | first = first(end-3:end);  %year is last four digits
      | 
      | last = get_param(sys,'LastModifiedDate');
      | if isempty(last)
      |     last = datestr(now,'yyyy');
      | else
      |     last = last(end-3:end);
      | end
      | 
      | if strcmp(first,last)
      |     fprintf('%s -- Copyright %s Nexteer',NxtrConf,first)
      | else
      |     fprintf('%s -- %s%s- %s Nexteer',NxtrConf,char(169),first,last)
      | end

== system CM620A_MotAg0Meas/MotAg0Meas/MotAg0MeasInit1/Compute Correction Table/NVM Ok/Configure Coefficients ==
  note: This block is for simulation purposes only.
      |
      | The data in shadowed RAM is to be populated
      | by NVM handler
  CopyRight2 : Subsystem  Description=|  mask(Copyright Information){none=on}
      | Copyright info block.                                               
      |                                                                     
      | Place copyright information at the top of every subsystem in design.
      mask prompts: none "No parameters"
      mask help: Place copyright information at the top of every subsystem in design.
      mask Display:
      | NxtrConf = 'Nexteer Confidential';
      | 
      | sys = bdroot; %handle for the current model ("system")
      | first = get_param(sys,'Created');
      | first = first(end-3:end);  %year is last four digits
      | 
      | last = get_param(sys,'LastModifiedDate');
      | if isempty(last)
      |     last = datestr(now,'yyyy');
      | else
      |     last = last(end-3:end);
      | end
      | 
      | if strcmp(first,last)
      |     fprintf('%s -- Copyright %s Nexteer',NxtrConf,first)
      | else
      |     fprintf('%s -- %s%s- %s Nexteer',NxtrConf,char(169),first,last)
      | end
  Data Store Write : DataStoreWrite  DataStoreName=MotAg0CoeffTbl
  temporary harmonic coefficient holder : Constant  Value=[0 0 0.0199999995529651642 0 0 0 0 0 0 0 0 0 0 0 0 0 0 0 0 0 0 0 0 0 0 0]  OutDataTypeStr=single
  wires:
  temporary harmonic coefficient holder/1 -> Data Store Write/1

== system CM620A_MotAg0Meas/MotAg0Meas/MotAg0MeasInit1/Compute Correction Table/NVM Ok/CopyRight2 ==

== system CM620A_MotAg0Meas/MotAg0Meas/MotAg0MeasPer1/Process MotAg0 Angle/FltInj_u08/CopyRight2 ==

== system CM620A_MotAg0Meas/MotAg0Meas/MotAg0MeasPer1/Process MotAg0 Angle/Process MotAg0Raw/Atomic Subsystem1 ==
  InputBoolean : Inport  OutDataTypeStr=boolean
  If : If  IfExpression=u1 ~= 0
  Merge : Merge
  Output 0 : Subsystem  TreatAsAtomicUnit=on
  Output 1 : Subsystem  TreatAsAtomicUnit=on
  OutputNumber : Outport  OutDataTypeStr=uint8
  wires:
  InputBoolean/1 -> If/1
  If/1 -> Output 1/Action
  If/2 -> Output 0/Action
  Output 1/1(Out1) -> Merge/1
  Output 0/1(Out1) -> Merge/2
  Merge/1 -> OutputNumber/1

== system CM620A_MotAg0Meas/MotAg0Meas/MotAg0MeasPer1/Process MotAg0 Angle/Process MotAg0Raw/Atomic Subsystem2 ==
  InputBoolean : Inport  OutDataTypeStr=boolean
  If : If  IfExpression=u1 ~= 0
  Merge : Merge
  Output 0 : Subsystem  TreatAsAtomicUnit=on
  Output 1 : Subsystem  TreatAsAtomicUnit=on
  OutputNumber : Outport  OutDataTypeStr=uint8
  wires:
  InputBoolean/1 -> If/1
  If/1 -> Output 1/Action
  If/2 -> Output 0/Action
  Output 1/1(Out1) -> Merge/1
  Output 0/1(Out1) -> Merge/2
  Merge/1 -> OutputNumber/1

== system CM620A_MotAg0Meas/MotAg0Meas/MotAg0MeasPer1/Process MotAg0 Angle/Process MotAg0Raw/Atomic Subsystem3 ==
  InputBoolean : Inport  OutDataTypeStr=boolean
  If : If  IfExpression=u1 ~= 0
  Merge : Merge
  Output 0 : Subsystem  TreatAsAtomicUnit=on
  Output 1 : Subsystem  TreatAsAtomicUnit=on
  OutputNumber : Outport  OutDataTypeStr=uint8
  wires:
  Merge/1 -> OutputNumber/1
  Output 0/1(Out1) -> Merge/2
  Output 1/1(Out1) -> Merge/1
  If/2 -> Output 0/Action
  If/1 -> Output 1/Action
  InputBoolean/1 -> If/1

== system CM620A_MotAg0Meas/MotAg0Meas/MotAg0MeasPer1/Process MotAg0 Angle/Process MotAg0Raw/CopyRight2 ==

== system CM620A_MotAg0Meas/MotAg0Meas/MotAg0MeasPer2/MotAg0 Protocol Fault Operation/Atomic Subsystem/CopyRight2 ==

== system CM620A_MotAg0Meas/MotAg0Meas/MotAg0MeasPer2/MotAg0 Protocol Fault Operation/Atomic Subsystem/N Step ==
  Action Port : ActionPort  ActionType=else
  Constant3 : Constant  Value=MOTAG0PRTCLFLTPASSSTEP_CNT_U16
  CopyRight2 : Subsystem  Description=|  mask(Copyright Information){none=on}
      | Copyright info block.                                               
      |                                                                     
      | Place copyright information at the top of every subsystem in design.
      mask prompts: none "No parameters"
      mask help: Place copyright information at the top of every subsystem in design.
      mask Display:
      | NxtrConf = 'Nexteer Confidential';
      | 
      | sys = bdroot; %handle for the current model ("system")
      | first = get_param(sys,'Created');
      | first = first(end-3:end);  %year is last four digits
      | 
      | last = get_param(sys,'LastModifiedDate');
      | if isempty(last)
      |     last = datestr(now,'yyyy');
      | else
      |     last = last(end-3:end);
      | end
      | 
      | if strcmp(first,last)
      |     fprintf('%s -- Copyright %s Nexteer',NxtrConf,first)
      | else
      |     fprintf('%s -- %s%s- %s Nexteer',NxtrConf,char(169),first,last)
      | end
  NtcNr1 : simulink/Sources/Enumerated Constant  OutDataTypeStr=Enum: NtcSts1  Value=NtcSts1.NTCSTS_PREPASSD  SampleTime=inf
  NtcSts : Outport
  DebStep : Outport  Port=2
  wires:
  Constant3/1 -> DebStep/1
  NtcNr1/1 -> NtcSts/1

== system CM620A_MotAg0Meas/MotAg0Meas/MotAg0MeasPer2/MotAg0 Protocol Fault Operation/Atomic Subsystem/P Step ==
  Action Port : ActionPort  ActionType=then
  Constant3 : Constant  Value=MOTAG0PRTCLFLTFAILSTEP_CNT_U16
  CopyRight2 : Subsystem  Description=|  mask(Copyright Information){none=on}
      | Copyright info block.                                               
      |                                                                     
      | Place copyright information at the top of every subsystem in design.
      mask prompts: none "No parameters"
      mask help: Place copyright information at the top of every subsystem in design.
      mask Display:
      | NxtrConf = 'Nexteer Confidential';
      | 
      | sys = bdroot; %handle for the current model ("system")
      | first = get_param(sys,'Created');
      | first = first(end-3:end);  %year is last four digits
      | 
      | last = get_param(sys,'LastModifiedDate');
      | if isempty(last)
      |     last = datestr(now,'yyyy');
      | else
      |     last = last(end-3:end);
      | end
      | 
      | if strcmp(first,last)
      |     fprintf('%s -- Copyright %s Nexteer',NxtrConf,first)
      | else
      |     fprintf('%s -- %s%s- %s Nexteer',NxtrConf,char(169),first,last)
      | end
  NtcNr1 : simulink/Sources/Enumerated Constant  OutDataTypeStr=Enum: NtcSts1  Value=NtcSts1.NTCSTS_PREFAILD  SampleTime=inf
  NtcSts : Outport
  DebStep : Outport  Port=2
  wires:
  NtcNr1/1 -> NtcSts/1
  Constant3/1 -> DebStep/1

== system CM620A_MotAg0Meas/MotAg0Meas/MotAg0MeasPer2/MotAg0 Protocol Fault Operation/GetNtcQlfr/CopyRight2 ==

== system CM620A_MotAg0Meas/MotAg0Meas/MotAg0MeasPer2/MotAg0 Protocol Fault Operation/SetNtcSts/CopyRight2 ==

== system CM620A_MotAg0Meas/MotAg0Meas/MotAg0MeasPer2/MotAg0 Protocol Fault Operation/Subsystem/Atomic Subsystem1 ==
  InputBoolean : Inport  OutDataTypeStr=boolean
  If : If  IfExpression=u1 ~= 0
  Merge : Merge
  Output 0 : Subsystem  TreatAsAtomicUnit=on
  Output 1 : Subsystem  TreatAsAtomicUnit=on
  OutputNumber : Outport  OutDataTypeStr=uint8
  wires:
  InputBoolean/1 -> If/1
  If/1 -> Output 1/Action
  If/2 -> Output 0/Action
  Output 1/1(Out1) -> Merge/1
  Output 0/1(Out1) -> Merge/2
  Merge/1 -> OutputNumber/1

== system CM620A_MotAg0Meas/MotAg0Meas/MotAg0MeasPer2/MotAg0 Protocol Fault Operation/Subsystem/Atomic Subsystem2 ==
  InputBoolean : Inport  OutDataTypeStr=boolean
  If : If  IfExpression=u1 ~= 0
  Merge : Merge
  Output 0 : Subsystem  TreatAsAtomicUnit=on
  Output 1 : Subsystem  TreatAsAtomicUnit=on
  OutputNumber : Outport  OutDataTypeStr=uint8
  wires:
  Merge/1 -> OutputNumber/1
  Output 0/1(Out1) -> Merge/2
  Output 1/1(Out1) -> Merge/1
  If/2 -> Output 0/Action
  If/1 -> Output 1/Action
  InputBoolean/1 -> If/1

== system CM620A_MotAg0Meas/MotAg0Meas/MotAg0MeasPer2/MotAg0 Protocol Fault Operation/Subsystem/Atomic Subsystem3 ==
  InputBoolean : Inport  OutDataTypeStr=boolean
  If : If  IfExpression=u1 ~= 0
  Merge : Merge
  Output 0 : Subsystem  TreatAsAtomicUnit=on
  Output 1 : Subsystem  TreatAsAtomicUnit=on
  OutputNumber : Outport  OutDataTypeStr=uint8
  wires:
  InputBoolean/1 -> If/1
  If/1 -> Output 1/Action
  If/2 -> Output 0/Action
  Output 1/1(Out1) -> Merge/1
  Output 0/1(Out1) -> Merge/2
  Merge/1 -> OutputNumber/1

== system CM620A_MotAg0Meas/MotAg0Meas/MotAg0MeasPer2/MotAg0 Protocol Fault Operation/Subsystem/CopyRight2 ==

== system CM620A_MotAg0Meas/MotAg0Meas/MotAg0MeasPer2/Process ErrorReg and DieRevCtr/Process MotAg0RawErr/CopyRight2 ==
